simulink model "GenerateProcessData"  (R2020b)
settings: Solver=VariableStepAuto  StartTime=0.0  StopTime=100  RelTol=1e-3
libraries: simulink x2
settings Model: Creator=tmlouw  LastModifiedBy=tmlouw

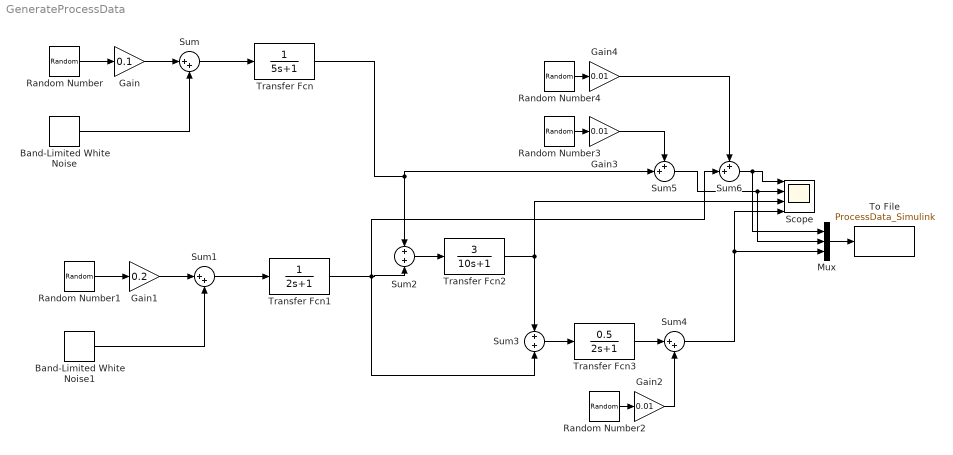
== system GenerateProcessData ==
  Band-Limited White Noise : simulink/Sources/Band-Limited White Noise  Cov=[0.1]  Ts=2  seed=[23341]
  Band-Limited White Noise1 : simulink/Sources/Band-Limited White Noise  Cov=[0.1]  Ts=2  seed=[23341]
  Gain : Gain  Gain=0.1
  Gain1 : Gain  Gain=0.2
  Gain2 : Gain  Gain=0.01
  Gain3 : Gain  Gain=0.01
  Gain4 : Gain  Gain=0.01
  Mux : Mux  Inputs=3
  Random Number{,1..4} (5 alike) : RandomNumber  SampleTime=0.1
  Scope : Scope  NumInputPorts=4
  Sum : Sum  Inputs=|++
  Sum1 : Sum  Inputs=|++
  Sum2 : Sum  Inputs=+|+
  Sum3 : Sum  Inputs=+|+
  Sum4 : Sum  Inputs=|++
  Sum5 : Sum  Inputs=++|
  Sum6 : Sum  Inputs=++|
  To File : ToFile  Filename=ProcessData_Simulink  MatrixName=Measurements  SaveFormat=Timeseries
  Transfer Fcn : TransferFcn  Denominator=[5 1]
  Transfer Fcn1 : TransferFcn  Denominator=[2 1]
  Transfer Fcn2 : TransferFcn  Numerator=[3]  Denominator=[10 1]
  Transfer Fcn3 : TransferFcn  Numerator=[0.5]  Denominator=[2 1]
  wires:
  Random Number/1 -> Gain/1
  Gain/1 -> Sum/1
  Band-Limited White Noise/1 -> Sum/2
  Sum/1 -> Transfer Fcn/1
  Transfer Fcn/1 -> Sum2/1, Sum5/2
  Gain1/1 -> Sum1/1
  Band-Limited White Noise1/1 -> Sum1/2
  Random Number1/1 -> Gain1/1
  Sum1/1 -> Transfer Fcn1/1
  Transfer Fcn1/1 -> Sum6/2, Sum3/2, Sum2/2
  Sum2/1 -> Transfer Fcn2/1
  Transfer Fcn2/1 -> Sum3/1, Scope/3
  Sum3/1 -> Transfer Fcn3/1
  Transfer Fcn3/1 -> Sum4/1
  Random Number2/1 -> Gain2/1
  Gain2/1 -> Sum4/2
  Random Number3/1 -> Gain3/1
  Random Number4/1 -> Gain4/1
  Gain3/1 -> Sum5/1
  Sum5/1 -> Mux/2, Scope/2
  Sum6/1 -> Mux/1, Scope/1
  Gain4/1 -> Sum6/1
  Mux/1 -> To File/1
  Sum4/1 -> Scope/4, Mux/3
